simulink model "andbot1dot2_voltage_loop_currectVersion"  (R2015b)
settings: Solver=VariableStepAuto  StartTime=0.0  StopTime=inf  RelTol=1e-3
values from neighbouring files (symbols this model uses):
  den = [1 1.7857]    [andbot1dot2_modeling_param.m]
  num = [0 1.6095]    [andbot1dot2_modeling_param.m]
  Tsample = 0.04    [andbot1dot2_modeling_param.m]    (also in andbot1dot2_param.m)
libraries: simulink x3, slctrlblks x1, cstblocks x1, simulink_extras x1
settings Model: Creator=shangwei  LastModifiedBy=root

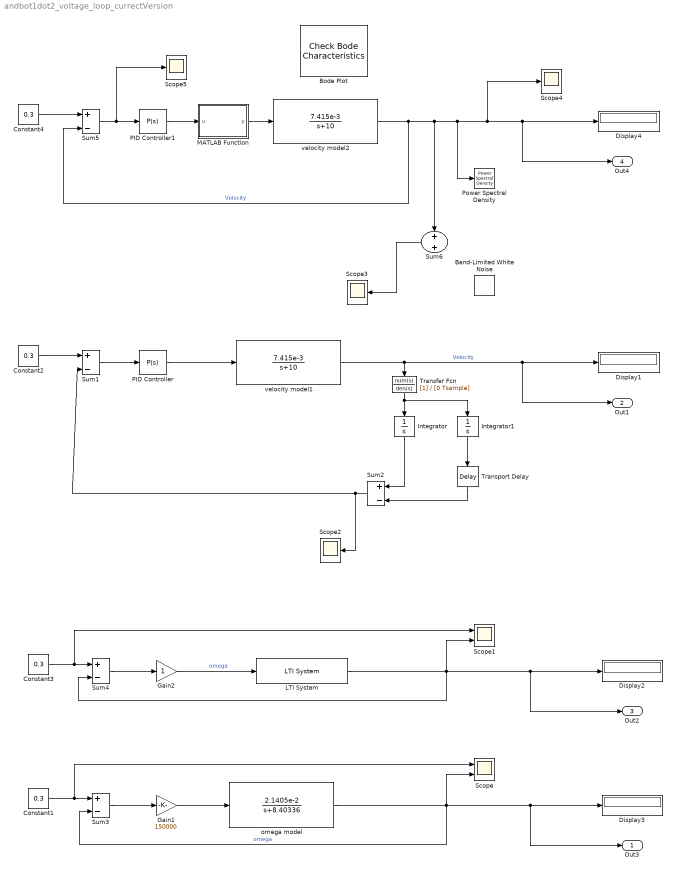
== system andbot1dot2_voltage_loop_currectVersion ==
  Band-Limited White Noise : simulink/Sources/Band-Limited White Noise  Cov=[0.5]  Ts=0.1  seed=[23341]
  Bode Plot : slctrlblks/Model Verification/Check Bode  Characteristics  InstantiateOnLoad=on  SaveOperatingPoints=off  LinearizationIOs={'/velocity model1', 1, 'outin', 'on', ''}  LinearizeAt=SnapshotTimes  SnapshotTimes=[0]  TriggerType=rising  SampleTime=auto  RateConversionMethod=zoh  PreWarpFreq=10  UseExactDelayModel=on  UseFullBlockNameLabels=off  UseBusSignalLabels=off  enabled=on  stopWhenAssertionFail=off  export=off  ViewDlgPos=[1726 281 540 424]  OpenViewOnLoad=on  LaunchViewOnOpen=on  FrequencyUnits=rad/s  MagnitudeUnits=dB  PhaseUnits=deg  TimeUnits=seconds  EnableUpperBound=off  UpperBoundFrequencies=[]  UpperBoundMagnitudes=[]  EnableLowerBound=off  LowerBoundFrequencies=[]  LowerBoundMagnitudes=[]
  Constant1 : Constant  Value=0.3
  Constant2 : Constant  Value=0.3
  Constant3 : Constant  Value=0.3
  Constant4 : Constant  Value=0.3  SampleTime=-1
  Display{1..4} (4 alike) : Display
  Gain1 : Gain  Gain=150000
  Gain2 : Gain
  Integrator : Integrator
  Integrator1 : Integrator
  LTI System : cstblocks/LTI System  sys=tf(num,den)  IC=[]
  MATLAB Function : MATLAB Function  TreatAsAtomicUnit=on
  PID Controller : simulink/Continuous/PID Controller  Controller=P  TimeDomain=Continuous-time  SampleTime=-1  IntegratorMethod=Forward Euler  FilterMethod=Forward Euler  Form=Parallel  UseFilter=on  ControllerParametersSource=internal  P=1  I=1  D=0  N=100  InitialConditionSource=internal  InitialConditionForIntegrator=0  InitialConditionForFilter=0  ExternalReset=none  LimitOutput=off  UpperSaturationLimit=inf  LowerSaturationLimit=-inf  LinearizeAsGain=on  AntiWindupMode=none  Kb=1  TrackingMode=off  Kt=1  PParamMin=[]  PParamMax=[]  IParamMin=[]  IParamMax=[]  DParamMin=[]  DParamMax=[]  NParamMin=[]  NParamMax=[]  KbParamMin=[]  KbParamMax=[]  KtParamMin=[]  KtParamMax=[]  POutMin=[]  POutMax=[]  IOutMin=[]  IOutMax=[]  DOutMin=[]  DOutMax=[]  NOutMin=[]  NOutMax=[]  KbOutMin=[]  KbOutMax=[]  KtOutMin=[]  KtOutMax=[]  IntegratorOutMin=[]  IntegratorOutMax=[]  FilterOutMin=[]  FilterOutMax=[]  SumOutMin=[]  SumOutMax=[]  SumI1OutMin=[]  SumI1OutMax=[]  SumI2OutMin=[]  SumI2OutMax=[]  SumI3OutMin=[]  SumI3OutMax=[]  SumDOutMin=[]  SumDOutMax=[]  SaturationOutMin=[]  SaturationOutMax=[]  IntegratorContinuousStateAttributes=''  IntegratorStateMustResolveToSignalObject=off  IntegratorRTWStateStorageClass=Auto  FilterContinuousStateAttributes=''  FilterStateMustResolveToSignalObject=off  FilterRTWStateStorageClass=Auto  DifferentiatorICPrevScaledInput=0  DifferentiatorOutMin=[]  DifferentiatorOutMax=[]
  PID Controller1 : simulink/Continuous/PID Controller  Controller=P  TimeDomain=Continuous-time  SampleTime=-1  IntegratorMethod=Forward Euler  FilterMethod=Forward Euler  Form=Parallel  UseFilter=on  ControllerParametersSource=internal  P=150000  I=1  D=0  N=100  InitialConditionSource=internal  InitialConditionForIntegrator=0  InitialConditionForFilter=0  ExternalReset=none  LimitOutput=off  UpperSaturationLimit=inf  LowerSaturationLimit=-inf  LinearizeAsGain=on  AntiWindupMode=none  Kb=1  TrackingMode=off  Kt=1  PParamMin=[]  PParamMax=[]  IParamMin=[]  IParamMax=[]  DParamMin=[]  DParamMax=[]  NParamMin=[]  NParamMax=[]  KbParamMin=[]  KbParamMax=[]  KtParamMin=[]  KtParamMax=[]  POutMin=[]  POutMax=[]  IOutMin=[]  IOutMax=[]  DOutMin=[]  DOutMax=[]  NOutMin=[]  NOutMax=[]  KbOutMin=[]  KbOutMax=[]  KtOutMin=[]  KtOutMax=[]  IntegratorOutMin=[]  IntegratorOutMax=[]  FilterOutMin=[]  FilterOutMax=[]  SumOutMin=[]  SumOutMax=[]  SumI1OutMin=[]  SumI1OutMax=[]  SumI2OutMin=[]  SumI2OutMax=[]  SumI3OutMin=[]  SumI3OutMax=[]  SumDOutMin=[]  SumDOutMax=[]  SaturationOutMin=[]  SaturationOutMax=[]  IntegratorContinuousStateAttributes=''  IntegratorStateMustResolveToSignalObject=off  IntegratorRTWStateStorageClass=Auto  FilterContinuousStateAttributes=''  FilterStateMustResolveToSignalObject=off  FilterRTWStateStorageClass=Auto  DifferentiatorICPrevScaledInput=0  DifferentiatorOutMin=[]  DifferentiatorOutMax=[]
  Power Spectral Density : simulink_extras/Additional Sinks/Power Spectral Density  npts=128  fftpts=512  HowOften=64  sampleT=0.1
  Scope : Scope  NumInputPorts=2
  Scope1 : Scope  NumInputPorts=2
  Scope{2..5} (4 alike) : Scope
  Sum{1..5} (5 alike) : Sum  Inputs=+-
  Sum6 : Sum
  Transfer Fcn : TransferFcn  Denominator=[0 Tsample]
  Transport Delay : TransportDelay  DelayTime=0.04
  omega model : TransferFcn  Numerator=[2.1405e-2]  Denominator=[1 8.40336]
  velocity model1 : TransferFcn  Numerator=[7.415e-3]  Denominator=[1 10]
  velocity model2 : TransferFcn  Numerator=[7.415e-3]  Denominator=[1 10]
  Out3 : Outport
  Out1 : Outport  Port=2
  Out2 : Outport  Port=3
  Out4 : Outport  Port=4
  wires:
  Sum3/1 -> Gain1/1
  omega model/1 -> Scope/2, Sum3/2, Out3/1, Display3/1  "omega"
  Constant1/1 -> Scope/1, Sum3/1
  Gain1/1 -> omega model/1
  Sum1/1 -> PID Controller/1
  velocity model1/1 -> Out1/1, Display1/1, Transfer Fcn/1  "Velocity"
  Constant2/1 -> Sum1/1
  PID Controller/1 -> velocity model1/1
  Integrator1/1 -> Transport Delay/1
  Integrator/1 -> Sum2/1
  Transport Delay/1 -> Sum2/2
  Sum2/1 -> Scope2/1, Sum1/2
  Sum4/1 -> Gain2/1
  Constant3/1 -> Sum4/1, Scope1/1
  LTI System/1 -> Sum4/2, Scope1/2, Display2/1, Out2/1
  Gain2/1 -> LTI System/1  "omega"
  Sum5/1 -> Scope5/1, PID Controller1/1
  velocity model2/1 -> Sum5/2, Sum6/1, Power Spectral Density/1, Scope4/1, Display4/1, Out4/1  "Velocity"
  Constant4/1 -> Sum5/1
  PID Controller1/1 -> MATLAB Function/1(u)
  Sum6/1 -> Scope3/1
  Transfer Fcn/1 -> Integrator1/1, Integrator/1
  MATLAB Function/1(y) -> velocity model2/1

== matlab function andbot1dot2_voltage_loop_currectVersion/MATLAB Function ==
  data: u input; y output
function y = fcn(u)
%#codegen

if u >= 260 
    y = 260;
elseif u <= -260;
        y = -260;
else
    y = u;
end
